simulink model "envelope_real"  (R2017a)
settings: Solver=VariableStepAuto  StartTime=0.0  StopTime=10  RelTol=1e-3
values from neighbouring files (symbols this model uses):
  DC_Gain = (R1*RL)/(RV*(R1+R2+RL)+R1*(R2+RL))    (= 0.0237981913375)    [Frequency_calc.m]
  S1 = RV/RL + (RV*R2)/(RL*R1) + RV/R1 + R2/RL + 1    (= 42.02)    [Frequency_calc.m]
  S2 = C2*RV + (R2*C2*RV)/R1 + (R2*C1*RV)/RL + C1*RV    (= 0.1022)    [Frequency_calc.m]
  S3 = -1/(RV*R2*C2*C1)    (= -100000)    [Frequency_calc.m]
undefined symbols (not defined in the file or in its folder): DiscIntNeverNeededParam
settings Model: Creator=Andre  LastModifiedBy=Andre

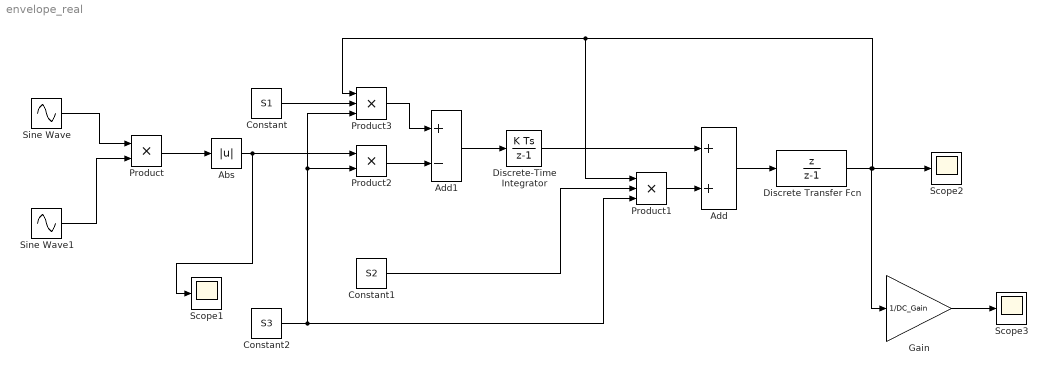
== system envelope_real ==
  Abs : Abs
  Add : Sum
  Add1 : Sum  Inputs=+-
  Constant : Constant  Value=S1
  Constant1 : Constant  Value=S2
  Constant2 : Constant  Value=S3
  Discrete Transfer Fcn : DiscreteTransferFcn  Numerator=[1 0]  Denominator=[1 -1]
  Discrete-Time Integrator : DiscreteIntegrator  InitialConditionSetting=State (most efficient)  SampleTime=-1  ICPrevOutput=DiscIntNeverNeededParam  ICPrevScaledInput=DiscIntNeverNeededParam
  Gain : Gain  Gain=1/DC_Gain
  Product : Product
  Product1 : Product  Inputs=***
  Product2 : Product
  Product3 : Product  Inputs=***
  Scope1 : Scope
  Scope2 : Scope
  Scope3 : Scope
  Sine Wave : Sin  Frequency=100000  SampleTime=0
  Sine Wave1 : Sin  SampleTime=0
  wires:
  Product/1 -> Abs/1
  Sine Wave/1 -> Product/1
  Sine Wave1/1 -> Product/2
  Discrete Transfer Fcn/1 -> Gain/1, Product3/1, Product1/1, Scope2/1
  Constant2/1 -> Product3/3, Product2/2, Product1/3
  Constant1/1 -> Product1/2
  Add/1 -> Discrete Transfer Fcn/1
  Product1/1 -> Add/2
  Discrete-Time Integrator/1 -> Add/1
  Add1/1 -> Discrete-Time Integrator/1
  Product3/1 -> Add1/1
  Product2/1 -> Add1/2
  Constant/1 -> Product3/2
  Abs/1 -> Scope1/1, Product2/1
  Gain/1 -> Scope3/1
